simulink model "RCAM_simulation_trim_temp"  (R2021b)
settings: Solver=VariableStepAuto  StartTime=0.0  StopTime=TF  FixedStep=0.0001  RelTol=1e-3
undefined symbols (not defined in the file): h0, lat0, lon0, RCAM_model, x0
libraries: aerolibfltsims x2
settings Model: Creator=khanh  LastModifiedBy=khanh

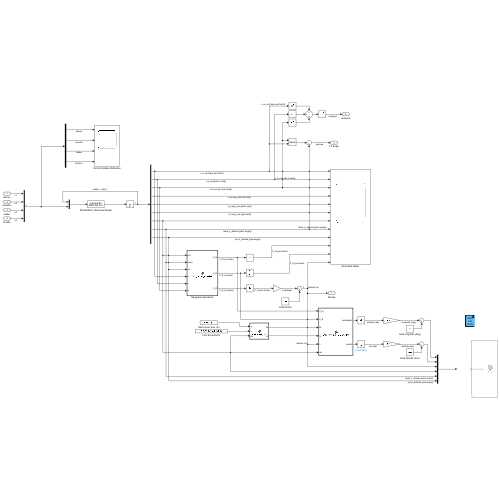
[thumbnail: Simulink's stored preview of the top-level diagram]
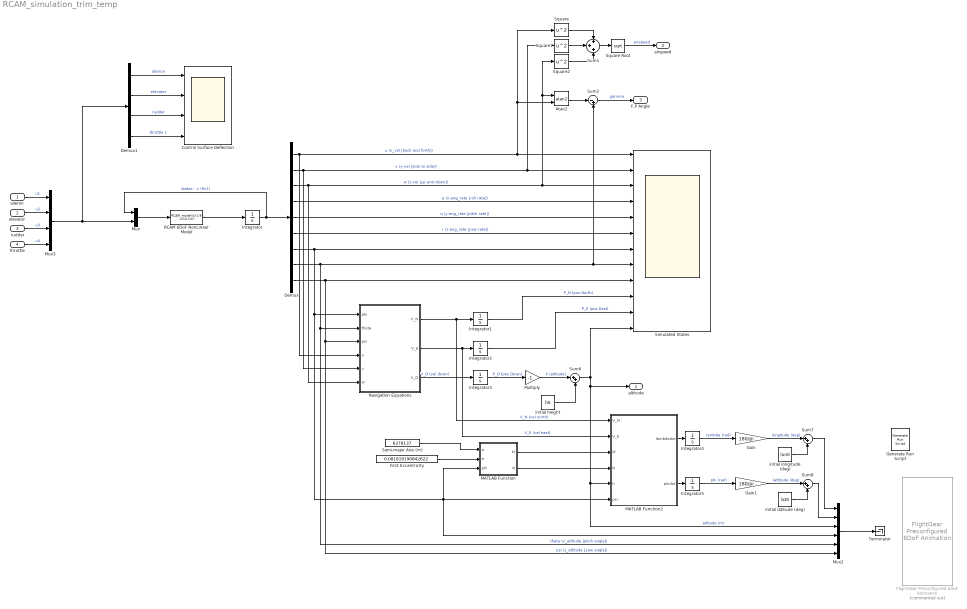
== system RCAM_simulation_trim_temp ==
  aileron : Inport
  elevator : Inport  Port=2
  rudder : Inport  Port=3
  throttle : Inport  Port=4
  Atan2 : Trigonometry  Operator=atan2
  Control Surface Deflection : Scope  NumInputPorts=4
  Demux : Demux  Outputs=9
  Demux1 : Demux
  First Eccentricity : Constant  Value=0.081819190842622
  FlightGear Preconfigured 6DoF Animation : aerolibfltsims/FlightGear Preconfigured 6DoF Animation  Commented=on  xFlightGearVersion=v2019.1  DestinationIpAddress=127.0.0.1  DestinationPort=5502  SampleTime=1/30  packetVersion=24
  Gain : Gain  Gain=180/pi
  Gain1 : Gain  Gain=180/pi
  Generate Run Script : aerolibfltsims/Generate Run Script  Architecture=Win64  dataFlow=Send  GeometryModelName=c172p  AirportId=KSFO  RunwayId=10L  InitialAltitude=7224  InitialHeading=113  OffsetDistance=4.72  OffsetAzimuth=0  InstallScenery=off  DisableShaders=on  OriginAddress=127.0.0.1  DestinationPort=5502  OriginPort=5505  LocalAddress=127.0.0.1  OutputFileName=runfg.bat  FlightGearBaseDirectory=C:\Program Files\FlightGear 2020.3
  Integrator : Integrator  InitialCondition=x0
  Integrator1 : Integrator  ContinuousStateAttributes='pos_north'
  Integrator2 : Integrator  ContinuousStateAttributes='pos_east'
  Integrator3 : Integrator  ContinuousStateAttributes='pos_down'
  Integrator4 : Integrator  ContinuousStateAttributes='lambda'
  Integrator5 : Integrator  UpperSaturationLimit=pi  LowerSaturationLimit=-pi  ContinuousStateAttributes='phi'
  MATLAB Function : MATLAB Function  TreatAsAtomicUnit=on
  MATLAB Function2 : MATLAB Function  TreatAsAtomicUnit=on
  Multiply : Gain  Gain=-1
  Mux : Mux  Inputs=2
  Mux2 : Mux  Inputs=6
  Mux3 : Mux
  Navigation Equations : MATLAB Function  TreatAsAtomicUnit=on
  RCAM 6DoF NonLinear Model : MATLABFcn  MATLABFcn=RCAM_model(u(1:9), u(10:13))
  Semi-major Axis (m) : Constant  Value=6378137
  Simulated States : Scope  NumInputPorts=12
  Square : Math  Operator=square  SaturateOnIntegerOverflow=on
  Square Root : Sqrt  SaturateOnIntegerOverflow=on
  Square1 : Math  Operator=square  SaturateOnIntegerOverflow=on
  Square2 : Math  Operator=square  SaturateOnIntegerOverflow=on
  Sum1 : Sum  Inputs=+++
  Sum2 : Sum  Inputs=|-+
  Sum6 : Sum  Inputs=|++
  Sum7 : Sum  Inputs=|++
  Sum8 : Sum  Inputs=|++
  Terminator : Terminator
  initial height : Constant  Value=h0
  initial latitude (deg) : Constant  Value=lat0
  initial longitude (deg) : Constant  Value=lon0
  altitude : Outport
  airspeed : Outport  Port=2
  F.P Angle : Outport  Port=3
  wires:
  RCAM 6DoF NonLinear Model/1 -> Integrator/1
  Integrator/1 -> Demux/1, Mux/1  "states - x (9x1)"
  Mux/1 -> RCAM 6DoF NonLinear Model/1
  Mux3/1 -> Demux1/1, Mux/2
  Demux1/1 -> Control Surface Deflection/1  "aileron"
  Demux1/2 -> Control Surface Deflection/2  "elevator"
  Demux1/3 -> Control Surface Deflection/3  "rudder"
  Demux1/4 -> Control Surface Deflection/4  "throttle 1"
  Demux/4 -> Simulated States/4  "p (x-ang_rate [roll rate])"
  Demux/5 -> Simulated States/5  "q (y-ang_rate [pitch rate])"
  Demux/6 -> Simulated States/6  "r (z-ang_rate [yaw rate])"
  Demux/9 -> Mux2/6, Navigation Equations/3(psi), Simulated States/9  "psi (z_attitude [yaw angle])"
  Navigation Equations/3(V_D) -> Integrator3/1  "V_D (vel down)"
  Navigation Equations/2(V_E) -> Integrator2/1, MATLAB Function2/2(V_E)  "V_E (vel east)"
  Navigation Equations/1(V_N) -> MATLAB Function2/1(V_N), Integrator1/1  "V_N (vel north)"
  Integrator1/1 -> Simulated States/10  "P_N (pos North)"
  Integrator2/1 -> Simulated States/11  "P_E (pos East)"
  Integrator3/1 -> Multiply/1  "P_D (pos Down)"
  Semi-major Axis (m)/1 -> MATLAB Function/1(a)
  First Eccentricity/1 -> MATLAB Function/2(e)
  MATLAB Function/2(N) -> MATLAB Function2/4(N)
  MATLAB Function/1(M) -> MATLAB Function2/3(M)
  Demux/7 -> MATLAB Function2/6(psi), MATLAB Function/3(phi), Mux2/4, Navigation Equations/1(phi), Simulated States/7
  Integrator5/1 -> Gain1/1  "phi (rad)"
  Integrator4/1 -> Gain/1  "lambda (rad)"
  Gain/1 -> Sum7/1  "longitude (deg)"
  Multiply/1 -> Sum6/1  "h (altitude)"
  Sum6/1 -> altitude/1, Mux2/3, MATLAB Function2/5(h), Simulated States/12  "altitude (m)"
  initial height/1 -> Sum6/2
  MATLAB Function2/1(lambdadot) -> Integrator4/1
  MATLAB Function2/2(phidot) -> Integrator5/1
  Gain1/1 -> Sum8/1  "lattitude (deg)"
  initial longitude (deg)/1 -> Sum7/2
  initial latitude (deg)/1 -> Sum8/2
  Sum7/1 -> Mux2/1
  Sum8/1 -> Mux2/2
  Mux2/1 -> Terminator/1
  aileron/1 -> Mux3/1  "u1"
  throttle/1 -> Mux3/4  "u4"
  rudder/1 -> Mux3/3  "u3"
  elevator/1 -> Mux3/2  "u2"
  Sum2/1 -> F.P Angle/1  "gamma"
  Atan2/1 -> Sum2/1
  Square Root/1 -> airspeed/1  "airspeed"
  Demux/1 -> Navigation Equations/4(u), Square/1, Atan2/2, Simulated States/1  "u (x_vel [back and forth])"
  Demux/2 -> Navigation Equations/5(v), Square1/1, Simulated States/2  "v (y-vel [side to side])"
  Square1/1 -> Sum1/2
  Square2/1 -> Sum1/3
  Demux/3 -> Navigation Equations/6(w), Square2/1, Atan2/1, Simulated States/3  "w (z-vel [up and down])"
  Square/1 -> Sum1/1
  Demux/8 -> Mux2/5, Navigation Equations/2(theta), Simulated States/8, Sum2/2  "theta (y_attitude [pitch angle])"
  Sum1/1 -> Square Root/1

== matlab function RCAM_simulation_trim_temp/MATLAB Function ==
  data: a input; M output; e input; phi input; N output
function [M, N] = calculate_mn (a, e, phi)

M = a*(1-e^2)/(1-(e^2)*sin(phi)^2)^1.5;

N = a/(1-(e^2)*sin(phi)^2)^0.5;

end

== matlab function RCAM_simulation_trim_temp/Navigation Equations ==
  data: phi input; theta input; psi input; u input; V_N output; v input; w input; V_E output; V_D output
function [V_N, V_E, V_D] = navigation_equation(phi, theta, psi, u, v, w)

x7 = phi;
x8 = theta;
x9 = psi;
x1 = u;
x2 = v;
x3 = w;

V_b = [x1; x2; x3];

%navigation equations
C1v = [cos(x9) sin(x9) 0; -sin(x9) cos(x9) 0; 0 0 1];

C21 = [cos(x8) 0 -sin(x8); 0 1 0; sin(x8) 0 cos(x8)];

Cb2 = [1 0 0; 0 cos(x7) sin(x7); 0 -sin(x7) cos(x7)];

Cvb = Cb2*C21*C1v;
Cvb = Cvb';

vel_vector = Cvb*V_b;

V_N = vel_vector(1);
V_E = vel_vector(2);
V_D = vel_vector(3);

end

== matlab function RCAM_simulation_trim_temp/MATLAB Function2 ==
  data: lambdadot output; V_N input; V_E input; phidot output; M input; N input; h input; psi input
function [lambdadot, phidot] = calculate_phi_lambdadot(V_N, V_E, M, N, h, psi)

lambdadot = V_E/(N+h)*cos(psi);
phidot = V_N/(M+h);


end
